simulink model "test_TFOIDFF"  (R2024a)
settings: Solver=VariableStepAuto  StartTime=0.0  StopTime=0.5  RelTol=1e-3
values from neighbouring files (symbols this model uses):
  loadedData = struct()    [colectare_TFOIDFF_simulink.m]
undefined symbols (not defined in the file or in its folder): control_a, control_p, force_a, force_p, minreal, oustapp, rpm_a, rpm_p
libraries: fod x146, slpidlib x15, cstblocks x9
(part 3 of 3)

== system test_TFOIDFF/TFOIDFFID/sensibility/Ord 9 H2 ==
  ref : Inport
  Fractional operator1 : fod/Fractional operator  Tag=Fractional operator  K=96.5  gam=0.99503  ww=[0.001, 1000]  n=7
      settings: SourceProductName=FOMCON Toolbox
  Fractional operator2 : fod/Fractional operator  Tag=Fractional operator  K=-59.619  gam=0.68457  ww=[0.001, 1000]  n=7
      settings: SourceProductName=FOMCON Toolbox
  Fractional operator3 : fod/Fractional operator  Tag=Fractional operator  K=1.4943  gam=0.49298  ww=[0.001, 1000]  n=7
      settings: SourceProductName=FOMCON Toolbox
  Fractional operator4 : fod/Fractional operator  Tag=Fractional operator  K=33.301  gam=0.42823  ww=[0.001, 1000]  n=7
      settings: SourceProductName=FOMCON Toolbox
  Fractional operator5 : fod/Fractional operator  Tag=Fractional operator  K=-67.092  gam=0.40076  ww=[0.001, 1000]  n=7
      settings: SourceProductName=FOMCON Toolbox
  Fractional operator6 : fod/Fractional operator  Tag=Fractional operator  K=55.242  gam=0.29512  ww=[0.001, 1000]  n=7
      settings: SourceProductName=FOMCON Toolbox
  Fractional operator7 : fod/Fractional operator  Tag=Fractional operator  K=53.481  gam=0.25349  ww=[0.001, 1000]  n=7
      settings: SourceProductName=FOMCON Toolbox
  Fractional operator8 : fod/Fractional operator  Tag=Fractional operator  K=42.107  gam=0.15698  ww=[0.001, 1000]  n=7
      settings: SourceProductName=FOMCON Toolbox
  Fractional operator9 : fod/Fractional operator  Tag=Fractional operator  K=-36.49  gam=0.039094  ww=[0.001, 1000]  n=7
      settings: SourceProductName=FOMCON Toolbox
  Sum : Sum  Inputs=|++++++
  Sum1 : Sum  Inputs=|+++
  Sum2 : Sum  Inputs=|++
  comanda : Outport
  wires:
  Sum/1 -> Sum2/1
  ref/1 -> Fractional operator1/1, Fractional operator2/1, Fractional operator9/1, Fractional operator8/1, Fractional operator7/1, Fractional operator6/1, Fractional operator5/1, Fractional operator4/1, Fractional operator3/1
  Fractional operator1/1 -> Sum/1
  Fractional operator2/1 -> Sum/2
  Fractional operator3/1 -> Sum/3
  Fractional operator4/1 -> Sum/4
  Fractional operator5/1 -> Sum/5
  Fractional operator6/1 -> Sum/6
  Fractional operator7/1 -> Sum1/1
  Fractional operator8/1 -> Sum1/2
  Fractional operator9/1 -> Sum1/3
  Sum1/1 -> Sum2/2
  Sum2/1 -> comanda/1

== system test_TFOIDFF/TFOIDFFID/sensibility/Regulator H22 ISE1 ==
  ref : Inport
  Ord 3 : Subsystem
  comanda : Outport
  wires:
  ref/1 -> Ord 3/1(ref)

== system test_TFOIDFF/TFOIDFFID/sensibility/Subsystem ==
  Reg_pitch : Inport
  In2 : Inport  Port=2
  Reg_azimuth : Inport  Port=3
  Azimuth H22 : Gain
  Comanda : Scope  NumInputPorts=3
  Comanda Iesire regulator : Scope  NumInputPorts=2
  D12 : TransferFcn  Numerator=[0.0019343*1 0.0019343*1.287]  Denominator=[1 1.322]
  D21 : TransferFcn  Numerator="[0.0014712*1    0.0014712*3.527]"  Denominator=[1 5.675]
  Pitch H11 : Gain
  Saturation5 : Saturate  UpperLimit=1  LowerLimit=-1  RndMeth=Ceiling
  Saturation6 : Saturate  UpperLimit=1  LowerLimit=-1  RndMeth=Ceiling
  Sum14 : Sum  Inputs=|++
  Sum16 : Sum  Inputs=|++
  TRAS 2_dof model 3 : Subsystem
  azimuth rpm : Outport
  azimuth pos : Outport  Port=2
  pitch rpm : Outport  Port=3
  Comanda1 : Outport  Port=4
  pitch pos : Outport  Port=5
  Comanda2 : Outport  Port=6
  wires:
  TRAS 2_dof model 3/3(rpm_p) -> pitch rpm/1  "pitch rpm"
  Saturation5/1 -> Pitch H11/1  "U_reg_Pitch"
  Azimuth H22/1 -> TRAS 2_dof model 3/1(ctr_a), Comanda1/1  "Comanda"
  TRAS 2_dof model 3/4(pos_p) -> pitch pos/1  "pitch pos"
  Sum14/1 -> Saturation5/1, Comanda Iesire regulator/1  "Pitch"
  Reg_azimuth/1 -> D12/1, Comanda/2, Sum16/2
  Saturation6/1 -> Azimuth H22/1  "U_reg_azimuth"
  TRAS 2_dof model 3/2(pos_a) -> azimuth pos/1  "azimuth pos"
  Pitch H11/1 -> TRAS 2_dof model 3/2(ctr_p), Comanda2/1  "Comanda"
  D12/1 -> Sum14/2
  In2/1 -> Comanda/3
  Sum16/1 -> Saturation6/1, Comanda Iesire regulator/2  "Azimuth"
  Reg_pitch/1 -> D21/1, Sum14/1, Comanda/1
  D21/1 -> Sum16/1
  TRAS 2_dof model 3/1(rpm_a) -> azimuth rpm/1  "azimuth rpm"

== system test_TFOIDFF/TFOIDFFID/IAE/Regulator H22 ISE1/Ord 3 ==
  ref : Inport
  Fractional operator1 : fod/Fractional operator  Tag=Fractional operator  K=97.313  gam=0.98233  ww=[0.001, 1000]  n=7
      settings: SourceProductName=FOMCON Toolbox
  Fractional operator2 : fod/Fractional operator  Tag=Fractional operator  K=44.439  gam=0.76232  ww=[0.001, 1000]  n=7
      settings: SourceProductName=FOMCON Toolbox
  Fractional operator3 : fod/Fractional operator  Tag=Fractional operator  K=-23.784  gam=0.61516  ww=[0.001, 1000]  n=7
      settings: SourceProductName=FOMCON Toolbox
  Sum : Sum  Inputs=+|++
  comanda : Outport
  wires:
  Sum/1 -> comanda/1
  ref/1 -> Fractional operator1/1, Fractional operator2/1, Fractional operator3/1
  Fractional operator1/1 -> Sum/1
  Fractional operator2/1 -> Sum/2
  Fractional operator3/1 -> Sum/3

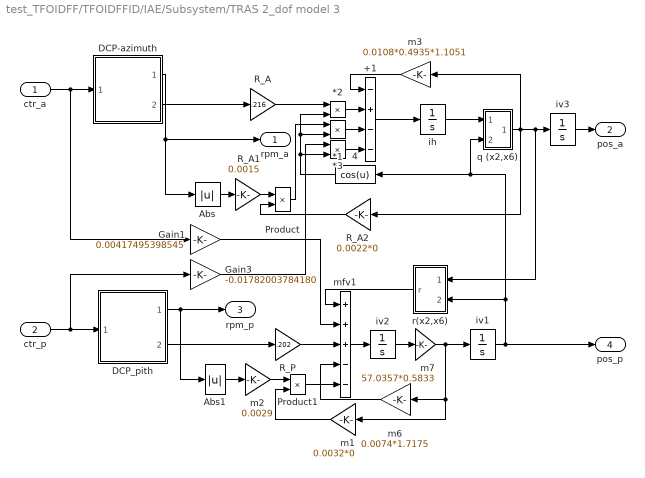
== system test_TFOIDFF/TFOIDFFID/IAE/Subsystem/TRAS 2_dof model 3 ==
  ctr_a : Inport
  ctr_p : Inport  Port=2
  *1 : Product  InputSameDT=on  SaturateOnIntegerOverflow=on  OutDataTypeStr=Inherit: Same as first input
  *2 : Product  InputSameDT=on  SaturateOnIntegerOverflow=on  OutDataTypeStr=Inherit: Same as first input
  *3 : Product  InputSameDT=on  SaturateOnIntegerOverflow=on  OutDataTypeStr=Inherit: Same as first input
  +1 : Sum  Inputs=-+--  InputSameDT=on  SaturateOnIntegerOverflow=on  OutDataTypeStr=Inherit: Same as first input
  4 : Fcn  Expr=cos(u)
  Abs : Abs
  Abs1 : Abs
  DCP-azimuth : Subsystem
  DCP_pith : Subsystem
  Gain1 : Gain  Gain=0.00417495398545  SaturateOnIntegerOverflow=on  OutDataTypeStr=Inherit: Same as input  ParamDataTypeStr=Inherit: Same as input
  Gain3 : Gain  Gain=-0.01782003784180  SaturateOnIntegerOverflow=on  OutDataTypeStr=Inherit: Same as input  ParamDataTypeStr=Inherit: Same as input
  Product : Product  InputSameDT=on  SaturateOnIntegerOverflow=on  OutDataTypeStr=Inherit: Same as first input
  Product1 : Product  SaturateOnIntegerOverflow=on  OutDataTypeStr=Inherit: Same as first input
  R_A : Gain  Gain=.216  OutDataTypeStr=Inherit: Same as input  ParamDataTypeStr=Inherit: Same as input
  R_A1 : Gain  Gain=0.0015  OutDataTypeStr=Inherit: Same as input  ParamDataTypeStr=Inherit: Same as input
  R_A2 : Gain  Gain=0.0022*0  OutDataTypeStr=Inherit: Same as input  ParamDataTypeStr=Inherit: Same as input
  R_P : Gain  Gain=.202  OutDataTypeStr=Inherit: Same as input  ParamDataTypeStr=Inherit: Same as input
  ih : Integrator  UpperSaturationLimit=10  LowerSaturationLimit=-10
  iv1 : Integrator  LimitOutput=on  UpperSaturationLimit=pi/2  LowerSaturationLimit=-pi/2
  iv2 : Integrator  UpperSaturationLimit=pi  LowerSaturationLimit=-pi
  iv3 : Integrator  LimitOutput=on  UpperSaturationLimit=6  LowerSaturationLimit=-6
  m1 : Gain  Gain=0.0032*0  SaturateOnIntegerOverflow=on  OutDataTypeStr=Inherit: Same as input  ParamDataTypeStr=Inherit: Same as input
  m2 : Gain  Gain=0.0029  SaturateOnIntegerOverflow=on  OutDataTypeStr=Inherit: Same as input  ParamDataTypeStr=Inherit: Same as input
  m3 : Gain  Gain=0.0108*0.4935*1.1051  OutDataTypeStr=Inherit: Same as input  ParamDataTypeStr=Inherit: Same as input
  m6 : Gain  Gain=0.0074*1.7175  OutDataTypeStr=Inherit: Same as input  ParamDataTypeStr=Inherit: Same as input
  m7 : Gain  Gain=57.0357*0.5833  SaturateOnIntegerOverflow=on  OutDataTypeStr=Inherit: Same as input  ParamDataTypeStr=Inherit: Same as input
  mfv1 : Sum  Inputs=+++--  InputSameDT=on  SaturateOnIntegerOverflow=on  OutDataTypeStr=Inherit: Same as first input
  q (x2,x6) : Subsystem
  r(x2,x6) : Subsystem
  rpm_a : Outport
  pos_a : Outport  Port=2
  rpm_p : Outport  Port=3
  pos_p : Outport  Port=4
  wires:
  DCP-azimuth/1(RPM_A) -> Abs/1, rpm_a/1
  +1/1 -> ih/1
  iv3/1 -> pos_a/1
  ctr_p/1 -> Gain3/1, DCP_pith/1(CTR_P)
  ctr_a/1 -> Gain1/1, DCP-azimuth/1(CTR_A)
  Gain3/1 -> *3/1
  Gain1/1 -> mfv1/2
  4/1 -> *3/2, *1/2, *2/2
  Product/1 -> *1/1
  *3/1 -> +1/4
  m2/1 -> Product1/1
  m1/1 -> Product1/2
  iv1/1 -> q (x2,x6)/2(x6), 4/1, r(x2,x6)/2(x6), pos_p/1
  R_P/1 -> mfv1/3
  r(x2,x6)/1(r) -> mfv1/1
  Product1/1 -> mfv1/5
  Abs1/1 -> m2/1
  DCP_pith/1(RPM_P) -> rpm_p/1, Abs1/1
  m7/1 -> m6/1, m1/1, iv1/1
  mfv1/1 -> iv2/1
  iv2/1 -> m7/1
  m6/1 -> mfv1/4
  DCP_pith/2(FORCE_P) -> R_P/1
  R_A2/1 -> Product/2
  R_A1/1 -> Product/1
  Abs/1 -> R_A1/1
  R_A/1 -> *2/1
  q (x2,x6)/1(q) -> R_A2/1, m3/1, r(x2,x6)/1(y2), iv3/1
  ih/1 -> q (x2,x6)/1(x2)
  *2/1 -> +1/2
  m3/1 -> +1/1
  *1/1 -> +1/3
  DCP-azimuth/2(FORCE_A) -> R_A/1

== system test_TFOIDFF/TFOIDFFID/ISE/Regulator H22 ISE1/Ord 3 ==
  ref : Inport
  Fractional operator1 : fod/Fractional operator  Tag=Fractional operator  K=97.313  gam=0.98233  ww=[0.001, 1000]  n=7
      settings: SourceProductName=FOMCON Toolbox
  Fractional operator2 : fod/Fractional operator  Tag=Fractional operator  K=44.439  gam=0.76232  ww=[0.001, 1000]  n=7
      settings: SourceProductName=FOMCON Toolbox
  Fractional operator3 : fod/Fractional operator  Tag=Fractional operator  K=-23.784  gam=0.61516  ww=[0.001, 1000]  n=7
      settings: SourceProductName=FOMCON Toolbox
  Sum : Sum  Inputs=+|++
  comanda : Outport
  wires:
  Sum/1 -> comanda/1
  ref/1 -> Fractional operator1/1, Fractional operator2/1, Fractional operator3/1
  Fractional operator1/1 -> Sum/1
  Fractional operator2/1 -> Sum/2
  Fractional operator3/1 -> Sum/3

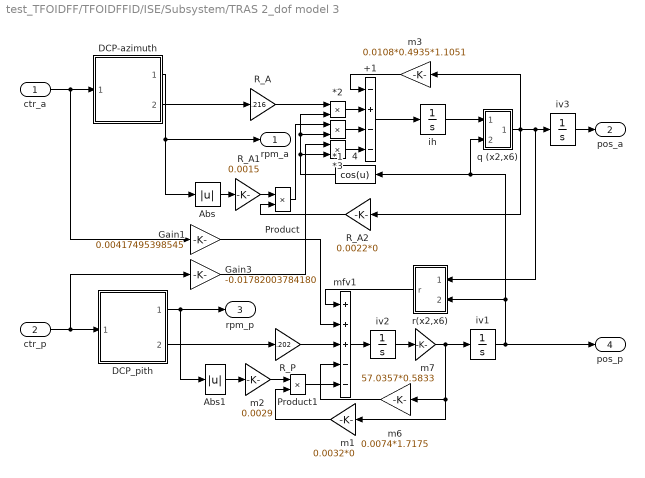
== system test_TFOIDFF/TFOIDFFID/ISE/Subsystem/TRAS 2_dof model 3 ==
  ctr_a : Inport
  ctr_p : Inport  Port=2
  *1 : Product  InputSameDT=on  SaturateOnIntegerOverflow=on  OutDataTypeStr=Inherit: Same as first input
  *2 : Product  InputSameDT=on  SaturateOnIntegerOverflow=on  OutDataTypeStr=Inherit: Same as first input
  *3 : Product  InputSameDT=on  SaturateOnIntegerOverflow=on  OutDataTypeStr=Inherit: Same as first input
  +1 : Sum  Inputs=-+--  InputSameDT=on  SaturateOnIntegerOverflow=on  OutDataTypeStr=Inherit: Same as first input
  4 : Fcn  Expr=cos(u)
  Abs : Abs
  Abs1 : Abs
  DCP-azimuth : Subsystem
  DCP_pith : Subsystem
  Gain1 : Gain  Gain=0.00417495398545  SaturateOnIntegerOverflow=on  OutDataTypeStr=Inherit: Same as input  ParamDataTypeStr=Inherit: Same as input
  Gain3 : Gain  Gain=-0.01782003784180  SaturateOnIntegerOverflow=on  OutDataTypeStr=Inherit: Same as input  ParamDataTypeStr=Inherit: Same as input
  Product : Product  InputSameDT=on  SaturateOnIntegerOverflow=on  OutDataTypeStr=Inherit: Same as first input
  Product1 : Product  SaturateOnIntegerOverflow=on  OutDataTypeStr=Inherit: Same as first input
  R_A : Gain  Gain=.216  OutDataTypeStr=Inherit: Same as input  ParamDataTypeStr=Inherit: Same as input
  R_A1 : Gain  Gain=0.0015  OutDataTypeStr=Inherit: Same as input  ParamDataTypeStr=Inherit: Same as input
  R_A2 : Gain  Gain=0.0022*0  OutDataTypeStr=Inherit: Same as input  ParamDataTypeStr=Inherit: Same as input
  R_P : Gain  Gain=.202  OutDataTypeStr=Inherit: Same as input  ParamDataTypeStr=Inherit: Same as input
  ih : Integrator  UpperSaturationLimit=10  LowerSaturationLimit=-10
  iv1 : Integrator  LimitOutput=on  UpperSaturationLimit=pi/2  LowerSaturationLimit=-pi/2
  iv2 : Integrator  UpperSaturationLimit=pi  LowerSaturationLimit=-pi
  iv3 : Integrator  LimitOutput=on  UpperSaturationLimit=6  LowerSaturationLimit=-6
  m1 : Gain  Gain=0.0032*0  SaturateOnIntegerOverflow=on  OutDataTypeStr=Inherit: Same as input  ParamDataTypeStr=Inherit: Same as input
  m2 : Gain  Gain=0.0029  SaturateOnIntegerOverflow=on  OutDataTypeStr=Inherit: Same as input  ParamDataTypeStr=Inherit: Same as input
  m3 : Gain  Gain=0.0108*0.4935*1.1051  OutDataTypeStr=Inherit: Same as input  ParamDataTypeStr=Inherit: Same as input
  m6 : Gain  Gain=0.0074*1.7175  OutDataTypeStr=Inherit: Same as input  ParamDataTypeStr=Inherit: Same as input
  m7 : Gain  Gain=57.0357*0.5833  SaturateOnIntegerOverflow=on  OutDataTypeStr=Inherit: Same as input  ParamDataTypeStr=Inherit: Same as input
  mfv1 : Sum  Inputs=+++--  InputSameDT=on  SaturateOnIntegerOverflow=on  OutDataTypeStr=Inherit: Same as first input
  q (x2,x6) : Subsystem
  r(x2,x6) : Subsystem
  rpm_a : Outport
  pos_a : Outport  Port=2
  rpm_p : Outport  Port=3
  pos_p : Outport  Port=4
  wires:
  DCP-azimuth/1(RPM_A) -> Abs/1, rpm_a/1
  +1/1 -> ih/1
  iv3/1 -> pos_a/1
  ctr_p/1 -> Gain3/1, DCP_pith/1(CTR_P)
  ctr_a/1 -> Gain1/1, DCP-azimuth/1(CTR_A)
  Gain3/1 -> *3/1
  Gain1/1 -> mfv1/2
  4/1 -> *3/2, *1/2, *2/2
  Product/1 -> *1/1
  *3/1 -> +1/4
  m2/1 -> Product1/1
  m1/1 -> Product1/2
  iv1/1 -> q (x2,x6)/2(x6), 4/1, r(x2,x6)/2(x6), pos_p/1
  R_P/1 -> mfv1/3
  r(x2,x6)/1(r) -> mfv1/1
  Product1/1 -> mfv1/5
  Abs1/1 -> m2/1
  DCP_pith/1(RPM_P) -> rpm_p/1, Abs1/1
  m7/1 -> m6/1, m1/1, iv1/1
  mfv1/1 -> iv2/1
  iv2/1 -> m7/1
  m6/1 -> mfv1/4
  DCP_pith/2(FORCE_P) -> R_P/1
  R_A2/1 -> Product/2
  R_A1/1 -> Product/1
  Abs/1 -> R_A1/1
  R_A/1 -> *2/1
  q (x2,x6)/1(q) -> R_A2/1, m3/1, r(x2,x6)/1(y2), iv3/1
  ih/1 -> q (x2,x6)/1(x2)
  *2/1 -> +1/2
  m3/1 -> +1/1
  *1/1 -> +1/3
  DCP-azimuth/2(FORCE_A) -> R_A/1

== system test_TFOIDFF/TFOIDFFID/ITAE/Regulator H22 ISE1/Ord 3 ==
  ref : Inport
  Fractional operator1 : fod/Fractional operator  Tag=Fractional operator  K=97.313  gam=0.98233  ww=[0.001, 1000]  n=7
      settings: SourceProductName=FOMCON Toolbox
  Fractional operator2 : fod/Fractional operator  Tag=Fractional operator  K=44.439  gam=0.76232  ww=[0.001, 1000]  n=7
      settings: SourceProductName=FOMCON Toolbox
  Fractional operator3 : fod/Fractional operator  Tag=Fractional operator  K=-23.784  gam=0.61516  ww=[0.001, 1000]  n=7
      settings: SourceProductName=FOMCON Toolbox
  Sum : Sum  Inputs=+|++
  comanda : Outport
  wires:
  Fractional operator3/1 -> Sum/3
  Fractional operator2/1 -> Sum/2
  Fractional operator1/1 -> Sum/1
  ref/1 -> Fractional operator3/1, Fractional operator2/1, Fractional operator1/1
  Sum/1 -> comanda/1

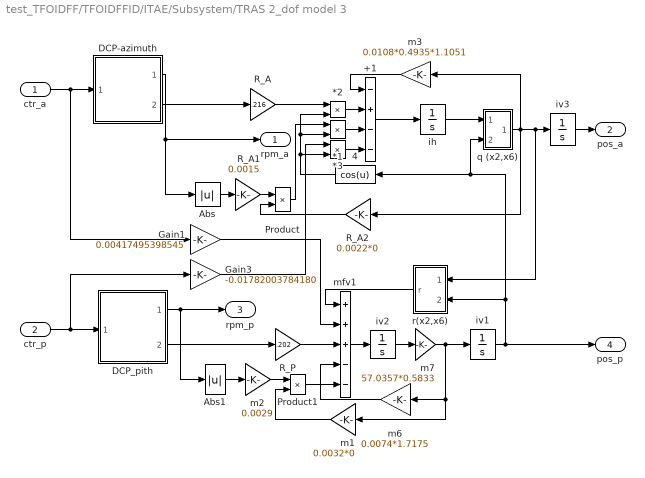
== system test_TFOIDFF/TFOIDFFID/ITAE/Subsystem/TRAS 2_dof model 3 ==
  ctr_a : Inport
  ctr_p : Inport  Port=2
  *1 : Product  InputSameDT=on  SaturateOnIntegerOverflow=on  OutDataTypeStr=Inherit: Same as first input
  *2 : Product  InputSameDT=on  SaturateOnIntegerOverflow=on  OutDataTypeStr=Inherit: Same as first input
  *3 : Product  InputSameDT=on  SaturateOnIntegerOverflow=on  OutDataTypeStr=Inherit: Same as first input
  +1 : Sum  Inputs=-+--  InputSameDT=on  SaturateOnIntegerOverflow=on  OutDataTypeStr=Inherit: Same as first input
  4 : Fcn  Expr=cos(u)
  Abs : Abs
  Abs1 : Abs
  DCP-azimuth : Subsystem
  DCP_pith : Subsystem
  Gain1 : Gain  Gain=0.00417495398545  SaturateOnIntegerOverflow=on  OutDataTypeStr=Inherit: Same as input  ParamDataTypeStr=Inherit: Same as input
  Gain3 : Gain  Gain=-0.01782003784180  SaturateOnIntegerOverflow=on  OutDataTypeStr=Inherit: Same as input  ParamDataTypeStr=Inherit: Same as input
  Product : Product  InputSameDT=on  SaturateOnIntegerOverflow=on  OutDataTypeStr=Inherit: Same as first input
  Product1 : Product  SaturateOnIntegerOverflow=on  OutDataTypeStr=Inherit: Same as first input
  R_A : Gain  Gain=.216  OutDataTypeStr=Inherit: Same as input  ParamDataTypeStr=Inherit: Same as input
  R_A1 : Gain  Gain=0.0015  OutDataTypeStr=Inherit: Same as input  ParamDataTypeStr=Inherit: Same as input
  R_A2 : Gain  Gain=0.0022*0  OutDataTypeStr=Inherit: Same as input  ParamDataTypeStr=Inherit: Same as input
  R_P : Gain  Gain=.202  OutDataTypeStr=Inherit: Same as input  ParamDataTypeStr=Inherit: Same as input
  ih : Integrator  UpperSaturationLimit=10  LowerSaturationLimit=-10
  iv1 : Integrator  LimitOutput=on  UpperSaturationLimit=pi/2  LowerSaturationLimit=-pi/2
  iv2 : Integrator  UpperSaturationLimit=pi  LowerSaturationLimit=-pi
  iv3 : Integrator  LimitOutput=on  UpperSaturationLimit=6  LowerSaturationLimit=-6
  m1 : Gain  Gain=0.0032*0  SaturateOnIntegerOverflow=on  OutDataTypeStr=Inherit: Same as input  ParamDataTypeStr=Inherit: Same as input
  m2 : Gain  Gain=0.0029  SaturateOnIntegerOverflow=on  OutDataTypeStr=Inherit: Same as input  ParamDataTypeStr=Inherit: Same as input
  m3 : Gain  Gain=0.0108*0.4935*1.1051  OutDataTypeStr=Inherit: Same as input  ParamDataTypeStr=Inherit: Same as input
  m6 : Gain  Gain=0.0074*1.7175  OutDataTypeStr=Inherit: Same as input  ParamDataTypeStr=Inherit: Same as input
  m7 : Gain  Gain=57.0357*0.5833  SaturateOnIntegerOverflow=on  OutDataTypeStr=Inherit: Same as input  ParamDataTypeStr=Inherit: Same as input
  mfv1 : Sum  Inputs=+++--  InputSameDT=on  SaturateOnIntegerOverflow=on  OutDataTypeStr=Inherit: Same as first input
  q (x2,x6) : Subsystem
  r(x2,x6) : Subsystem
  rpm_a : Outport
  pos_a : Outport  Port=2
  rpm_p : Outport  Port=3
  pos_p : Outport  Port=4
  wires:
  DCP-azimuth/2(FORCE_A) -> R_A/1
  *1/1 -> +1/3
  m3/1 -> +1/1
  *2/1 -> +1/2
  ih/1 -> q (x2,x6)/1(x2)
  q (x2,x6)/1(q) -> iv3/1, r(x2,x6)/1(y2), m3/1, R_A2/1
  R_A/1 -> *2/1
  Abs/1 -> R_A1/1
  R_A1/1 -> Product/1
  R_A2/1 -> Product/2
  DCP_pith/2(FORCE_P) -> R_P/1
  m6/1 -> mfv1/4
  iv2/1 -> m7/1
  mfv1/1 -> iv2/1
  m7/1 -> iv1/1, m1/1, m6/1
  DCP_pith/1(RPM_P) -> Abs1/1, rpm_p/1
  Abs1/1 -> m2/1
  Product1/1 -> mfv1/5
  r(x2,x6)/1(r) -> mfv1/1
  R_P/1 -> mfv1/3
  iv1/1 -> pos_p/1, r(x2,x6)/2(x6), 4/1, q (x2,x6)/2(x6)
  m1/1 -> Product1/2
  m2/1 -> Product1/1
  *3/1 -> +1/4
  Product/1 -> *1/1
  4/1 -> *2/2, *1/2, *3/2
  Gain1/1 -> mfv1/2
  Gain3/1 -> *3/1
  ctr_a/1 -> DCP-azimuth/1(CTR_A), Gain1/1
  ctr_p/1 -> DCP_pith/1(CTR_P), Gain3/1
  iv3/1 -> pos_a/1
  +1/1 -> ih/1
  DCP-azimuth/1(RPM_A) -> rpm_a/1, Abs/1

== system test_TFOIDFF/TFOIDFFID/ITSE/Regulator H22 ISE1/Ord 3 ==
  ref : Inport
  Fractional operator1 : fod/Fractional operator  Tag=Fractional operator  K=97.313  gam=0.98233  ww=[0.001, 1000]  n=7
      settings: SourceProductName=FOMCON Toolbox
  Fractional operator2 : fod/Fractional operator  Tag=Fractional operator  K=44.439  gam=0.76232  ww=[0.001, 1000]  n=7
      settings: SourceProductName=FOMCON Toolbox
  Fractional operator3 : fod/Fractional operator  Tag=Fractional operator  K=-23.784  gam=0.61516  ww=[0.001, 1000]  n=7
      settings: SourceProductName=FOMCON Toolbox
  Sum : Sum  Inputs=+|++
  comanda : Outport
  wires:
  Fractional operator3/1 -> Sum/3
  Fractional operator2/1 -> Sum/2
  Fractional operator1/1 -> Sum/1
  ref/1 -> Fractional operator3/1, Fractional operator2/1, Fractional operator1/1
  Sum/1 -> comanda/1

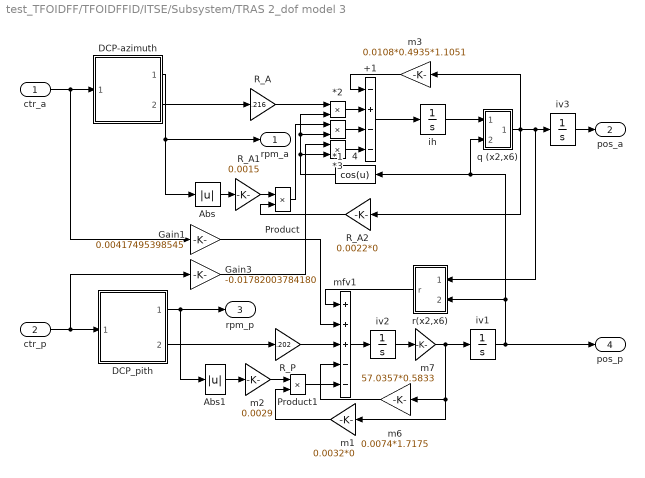
== system test_TFOIDFF/TFOIDFFID/ITSE/Subsystem/TRAS 2_dof model 3 ==
  ctr_a : Inport
  ctr_p : Inport  Port=2
  *1 : Product  InputSameDT=on  SaturateOnIntegerOverflow=on  OutDataTypeStr=Inherit: Same as first input
  *2 : Product  InputSameDT=on  SaturateOnIntegerOverflow=on  OutDataTypeStr=Inherit: Same as first input
  *3 : Product  InputSameDT=on  SaturateOnIntegerOverflow=on  OutDataTypeStr=Inherit: Same as first input
  +1 : Sum  Inputs=-+--  InputSameDT=on  SaturateOnIntegerOverflow=on  OutDataTypeStr=Inherit: Same as first input
  4 : Fcn  Expr=cos(u)
  Abs : Abs
  Abs1 : Abs
  DCP-azimuth : Subsystem
  DCP_pith : Subsystem
  Gain1 : Gain  Gain=0.00417495398545  SaturateOnIntegerOverflow=on  OutDataTypeStr=Inherit: Same as input  ParamDataTypeStr=Inherit: Same as input
  Gain3 : Gain  Gain=-0.01782003784180  SaturateOnIntegerOverflow=on  OutDataTypeStr=Inherit: Same as input  ParamDataTypeStr=Inherit: Same as input
  Product : Product  InputSameDT=on  SaturateOnIntegerOverflow=on  OutDataTypeStr=Inherit: Same as first input
  Product1 : Product  SaturateOnIntegerOverflow=on  OutDataTypeStr=Inherit: Same as first input
  R_A : Gain  Gain=.216  OutDataTypeStr=Inherit: Same as input  ParamDataTypeStr=Inherit: Same as input
  R_A1 : Gain  Gain=0.0015  OutDataTypeStr=Inherit: Same as input  ParamDataTypeStr=Inherit: Same as input
  R_A2 : Gain  Gain=0.0022*0  OutDataTypeStr=Inherit: Same as input  ParamDataTypeStr=Inherit: Same as input
  R_P : Gain  Gain=.202  OutDataTypeStr=Inherit: Same as input  ParamDataTypeStr=Inherit: Same as input
  ih : Integrator  UpperSaturationLimit=10  LowerSaturationLimit=-10
  iv1 : Integrator  LimitOutput=on  UpperSaturationLimit=pi/2  LowerSaturationLimit=-pi/2
  iv2 : Integrator  UpperSaturationLimit=pi  LowerSaturationLimit=-pi
  iv3 : Integrator  LimitOutput=on  UpperSaturationLimit=6  LowerSaturationLimit=-6
  m1 : Gain  Gain=0.0032*0  SaturateOnIntegerOverflow=on  OutDataTypeStr=Inherit: Same as input  ParamDataTypeStr=Inherit: Same as input
  m2 : Gain  Gain=0.0029  SaturateOnIntegerOverflow=on  OutDataTypeStr=Inherit: Same as input  ParamDataTypeStr=Inherit: Same as input
  m3 : Gain  Gain=0.0108*0.4935*1.1051  OutDataTypeStr=Inherit: Same as input  ParamDataTypeStr=Inherit: Same as input
  m6 : Gain  Gain=0.0074*1.7175  OutDataTypeStr=Inherit: Same as input  ParamDataTypeStr=Inherit: Same as input
  m7 : Gain  Gain=57.0357*0.5833  SaturateOnIntegerOverflow=on  OutDataTypeStr=Inherit: Same as input  ParamDataTypeStr=Inherit: Same as input
  mfv1 : Sum  Inputs=+++--  InputSameDT=on  SaturateOnIntegerOverflow=on  OutDataTypeStr=Inherit: Same as first input
  q (x2,x6) : Subsystem
  r(x2,x6) : Subsystem
  rpm_a : Outport
  pos_a : Outport  Port=2
  rpm_p : Outport  Port=3
  pos_p : Outport  Port=4
  wires:
  DCP-azimuth/2(FORCE_A) -> R_A/1
  *1/1 -> +1/3
  m3/1 -> +1/1
  *2/1 -> +1/2
  ih/1 -> q (x2,x6)/1(x2)
  q (x2,x6)/1(q) -> iv3/1, r(x2,x6)/1(y2), m3/1, R_A2/1
  R_A/1 -> *2/1
  Abs/1 -> R_A1/1
  R_A1/1 -> Product/1
  R_A2/1 -> Product/2
  DCP_pith/2(FORCE_P) -> R_P/1
  m6/1 -> mfv1/4
  iv2/1 -> m7/1
  mfv1/1 -> iv2/1
  m7/1 -> iv1/1, m1/1, m6/1
  DCP_pith/1(RPM_P) -> Abs1/1, rpm_p/1
  Abs1/1 -> m2/1
  Product1/1 -> mfv1/5
  r(x2,x6)/1(r) -> mfv1/1
  R_P/1 -> mfv1/3
  iv1/1 -> pos_p/1, r(x2,x6)/2(x6), 4/1, q (x2,x6)/2(x6)
  m1/1 -> Product1/2
  m2/1 -> Product1/1
  *3/1 -> +1/4
  Product/1 -> *1/1
  4/1 -> *2/2, *1/2, *3/2
  Gain1/1 -> mfv1/2
  Gain3/1 -> *3/1
  ctr_a/1 -> DCP-azimuth/1(CTR_A), Gain1/1
  ctr_p/1 -> DCP_pith/1(CTR_P), Gain3/1
  iv3/1 -> pos_a/1
  +1/1 -> ih/1
  DCP-azimuth/1(RPM_A) -> rpm_a/1, Abs/1

== system test_TFOIDFF/TFOIDFFID/sensibility/Regulator H22 ISE1/Ord 3 ==
  ref : Inport
  Fractional operator1 : fod/Fractional operator  Tag=Fractional operator  K=97.313  gam=0.98233  ww=[0.001, 1000]  n=7
      settings: SourceProductName=FOMCON Toolbox
  Fractional operator2 : fod/Fractional operator  Tag=Fractional operator  K=44.439  gam=0.76232  ww=[0.001, 1000]  n=7
      settings: SourceProductName=FOMCON Toolbox
  Fractional operator3 : fod/Fractional operator  Tag=Fractional operator  K=-23.784  gam=0.61516  ww=[0.001, 1000]  n=7
      settings: SourceProductName=FOMCON Toolbox
  Sum : Sum  Inputs=+|++
  comanda : Outport
  wires:
  Sum/1 -> comanda/1
  ref/1 -> Fractional operator1/1, Fractional operator2/1, Fractional operator3/1
  Fractional operator1/1 -> Sum/1
  Fractional operator2/1 -> Sum/2
  Fractional operator3/1 -> Sum/3

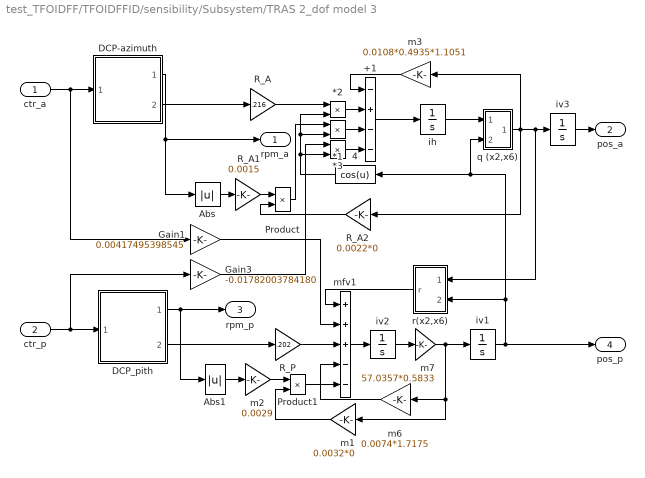
== system test_TFOIDFF/TFOIDFFID/sensibility/Subsystem/TRAS 2_dof model 3 ==
  ctr_a : Inport
  ctr_p : Inport  Port=2
  *1 : Product  InputSameDT=on  SaturateOnIntegerOverflow=on  OutDataTypeStr=Inherit: Same as first input
  *2 : Product  InputSameDT=on  SaturateOnIntegerOverflow=on  OutDataTypeStr=Inherit: Same as first input
  *3 : Product  InputSameDT=on  SaturateOnIntegerOverflow=on  OutDataTypeStr=Inherit: Same as first input
  +1 : Sum  Inputs=-+--  InputSameDT=on  SaturateOnIntegerOverflow=on  OutDataTypeStr=Inherit: Same as first input
  4 : Fcn  Expr=cos(u)
  Abs : Abs
  Abs1 : Abs
  DCP-azimuth : Subsystem
  DCP_pith : Subsystem
  Gain1 : Gain  Gain=0.00417495398545  SaturateOnIntegerOverflow=on  OutDataTypeStr=Inherit: Same as input  ParamDataTypeStr=Inherit: Same as input
  Gain3 : Gain  Gain=-0.01782003784180  SaturateOnIntegerOverflow=on  OutDataTypeStr=Inherit: Same as input  ParamDataTypeStr=Inherit: Same as input
  Product : Product  InputSameDT=on  SaturateOnIntegerOverflow=on  OutDataTypeStr=Inherit: Same as first input
  Product1 : Product  SaturateOnIntegerOverflow=on  OutDataTypeStr=Inherit: Same as first input
  R_A : Gain  Gain=.216  OutDataTypeStr=Inherit: Same as input  ParamDataTypeStr=Inherit: Same as input
  R_A1 : Gain  Gain=0.0015  OutDataTypeStr=Inherit: Same as input  ParamDataTypeStr=Inherit: Same as input
  R_A2 : Gain  Gain=0.0022*0  OutDataTypeStr=Inherit: Same as input  ParamDataTypeStr=Inherit: Same as input
  R_P : Gain  Gain=.202  OutDataTypeStr=Inherit: Same as input  ParamDataTypeStr=Inherit: Same as input
  ih : Integrator  UpperSaturationLimit=10  LowerSaturationLimit=-10
  iv1 : Integrator  LimitOutput=on  UpperSaturationLimit=pi/2  LowerSaturationLimit=-pi/2
  iv2 : Integrator  UpperSaturationLimit=pi  LowerSaturationLimit=-pi
  iv3 : Integrator  LimitOutput=on  UpperSaturationLimit=6  LowerSaturationLimit=-6
  m1 : Gain  Gain=0.0032*0  SaturateOnIntegerOverflow=on  OutDataTypeStr=Inherit: Same as input  ParamDataTypeStr=Inherit: Same as input
  m2 : Gain  Gain=0.0029  SaturateOnIntegerOverflow=on  OutDataTypeStr=Inherit: Same as input  ParamDataTypeStr=Inherit: Same as input
  m3 : Gain  Gain=0.0108*0.4935*1.1051  OutDataTypeStr=Inherit: Same as input  ParamDataTypeStr=Inherit: Same as input
  m6 : Gain  Gain=0.0074*1.7175  OutDataTypeStr=Inherit: Same as input  ParamDataTypeStr=Inherit: Same as input
  m7 : Gain  Gain=57.0357*0.5833  SaturateOnIntegerOverflow=on  OutDataTypeStr=Inherit: Same as input  ParamDataTypeStr=Inherit: Same as input
  mfv1 : Sum  Inputs=+++--  InputSameDT=on  SaturateOnIntegerOverflow=on  OutDataTypeStr=Inherit: Same as first input
  q (x2,x6) : Subsystem
  r(x2,x6) : Subsystem
  rpm_a : Outport
  pos_a : Outport  Port=2
  rpm_p : Outport  Port=3
  pos_p : Outport  Port=4
  wires:
  DCP-azimuth/1(RPM_A) -> Abs/1, rpm_a/1
  +1/1 -> ih/1
  iv3/1 -> pos_a/1
  ctr_p/1 -> Gain3/1, DCP_pith/1(CTR_P)
  ctr_a/1 -> Gain1/1, DCP-azimuth/1(CTR_A)
  Gain3/1 -> *3/1
  Gain1/1 -> mfv1/2
  4/1 -> *3/2, *1/2, *2/2
  Product/1 -> *1/1
  *3/1 -> +1/4
  m2/1 -> Product1/1
  m1/1 -> Product1/2
  iv1/1 -> q (x2,x6)/2(x6), 4/1, r(x2,x6)/2(x6), pos_p/1
  R_P/1 -> mfv1/3
  r(x2,x6)/1(r) -> mfv1/1
  Product1/1 -> mfv1/5
  Abs1/1 -> m2/1
  DCP_pith/1(RPM_P) -> rpm_p/1, Abs1/1
  m7/1 -> m6/1, m1/1, iv1/1
  mfv1/1 -> iv2/1
  iv2/1 -> m7/1
  m6/1 -> mfv1/4
  DCP_pith/2(FORCE_P) -> R_P/1
  R_A2/1 -> Product/2
  R_A1/1 -> Product/1
  Abs/1 -> R_A1/1
  R_A/1 -> *2/1
  q (x2,x6)/1(q) -> R_A2/1, m3/1, r(x2,x6)/1(y2), iv3/1
  ih/1 -> q (x2,x6)/1(x2)
  *2/1 -> +1/2
  m3/1 -> +1/1
  *1/1 -> +1/3
  DCP-azimuth/2(FORCE_A) -> R_A/1

== system test_TFOIDFF/TFOIDFFID/IAE/Subsystem/TRAS 2_dof model 3/DCP-azimuth ==
  CTR_A : Inport
  1/Ja : Gain  Gain=37000  SaturateOnIntegerOverflow=on  OutDataTypeStr=Inherit: Same as input  ParamDataTypeStr=Inherit: Same as input
  CtrlA(rpma) : Lookup  InputValues=rpm_a  Table=control_a
  Integrator1 : Integrator
  Sum1 : Sum  Inputs=|+-  InputSameDT=on  SaturateOnIntegerOverflow=on  OutDataTypeStr=Inherit: Same as first input
  forceA(rpma) : Lookup  InputValues=rpm_a  Table=force_a
  RPM_A : Outport
  FORCE_A : Outport  Port=2
  wires:
  forceA(rpma)/1 -> FORCE_A/1
  CTR_A/1 -> Sum1/1
  1/Ja/1 -> RPM_A/1, forceA(rpma)/1, CtrlA(rpma)/1
  Integrator1/1 -> 1/Ja/1
  CtrlA(rpma)/1 -> Sum1/2
  Sum1/1 -> Integrator1/1

== system test_TFOIDFF/TFOIDFFID/IAE/Subsystem/TRAS 2_dof model 3/DCP_pith ==
  CTR_P : Inport
  1/Jp1 : Gain  Gain=6100  OutDataTypeStr=Inherit: Same as input  ParamDataTypeStr=Inherit: Same as input
  CtrlP(rpmp) : Lookup  InputValues=rpm_p  Table=control_p
  Integrator : Integrator
  Sum : Sum  Inputs=|+-  InputSameDT=on  SaturateOnIntegerOverflow=on  OutDataTypeStr=Inherit: Same as first input
  force(rpmp) : Lookup  InputValues=rpm_p  Table=force_p
  RPM_P : Outport
  FORCE_P : Outport  Port=2
  wires:
  force(rpmp)/1 -> FORCE_P/1
  CTR_P/1 -> Sum/1
  1/Jp1/1 -> force(rpmp)/1, CtrlP(rpmp)/1, RPM_P/1
  CtrlP(rpmp)/1 -> Sum/2
  Integrator/1 -> 1/Jp1/1
  Sum/1 -> Integrator/1

== system test_TFOIDFF/TFOIDFFID/IAE/Subsystem/TRAS 2_dof model 3/q (x2,x6) ==
  x2 : Inport
  x6 : Inport  Port=2
  " q(x6)" : Fcn  Expr=( (0.0268-0.00300962066650)*cos(u)^2) +0.00300962066650
  *1 : Product  Inputs=*/  InputSameDT=on  SaturateOnIntegerOverflow=on  OutDataTypeStr=Inherit: Same as first input
  q : Outport
  wires:
  " q(x6)"/1 -> *1/2
  x6/1 -> " q(x6)"/1
  x2/1 -> *1/1
  *1/1 -> q/1

== system test_TFOIDFF/TFOIDFFID/IAE/Subsystem/TRAS 2_dof model 3/r(x2,x6) ==
  y2 : Inport
  x6 : Inport  Port=2
  +2 : Sum  InputSameDT=on  SaturateOnIntegerOverflow=on  OutDataTypeStr=Inherit: Same as first input
  Mux : Mux  Inputs=2
  r2 : Fcn  Expr=- ( 0.0292*cos(u)+ 0.0546*sin(u))*1.7143
  s : Fcn  Expr="(u(1)^2)*(     -0.07389953104162*  0.28753198180218*sin(u(2))*cos(u(2)))"
  r : Outport
  wires:
  y2/1 -> Mux/1
  +2/1 -> r/1
  x6/1 -> r2/1, Mux/2
  s/1 -> +2/2
  r2/1 -> +2/1
  Mux/1 -> s/1

== system test_TFOIDFF/TFOIDFFID/ISE/Subsystem/TRAS 2_dof model 3/DCP-azimuth ==
  CTR_A : Inport
  1/Ja : Gain  Gain=37000  SaturateOnIntegerOverflow=on  OutDataTypeStr=Inherit: Same as input  ParamDataTypeStr=Inherit: Same as input
  CtrlA(rpma) : Lookup  InputValues=rpm_a  Table=control_a
  Integrator1 : Integrator
  Sum1 : Sum  Inputs=|+-  InputSameDT=on  SaturateOnIntegerOverflow=on  OutDataTypeStr=Inherit: Same as first input
  forceA(rpma) : Lookup  InputValues=rpm_a  Table=force_a
  RPM_A : Outport
  FORCE_A : Outport  Port=2
  wires:
  forceA(rpma)/1 -> FORCE_A/1
  CTR_A/1 -> Sum1/1
  1/Ja/1 -> RPM_A/1, forceA(rpma)/1, CtrlA(rpma)/1
  Integrator1/1 -> 1/Ja/1
  CtrlA(rpma)/1 -> Sum1/2
  Sum1/1 -> Integrator1/1

== system test_TFOIDFF/TFOIDFFID/ISE/Subsystem/TRAS 2_dof model 3/DCP_pith ==
  CTR_P : Inport
  1/Jp1 : Gain  Gain=6100  OutDataTypeStr=Inherit: Same as input  ParamDataTypeStr=Inherit: Same as input
  CtrlP(rpmp) : Lookup  InputValues=rpm_p  Table=control_p
  Integrator : Integrator
  Sum : Sum  Inputs=|+-  InputSameDT=on  SaturateOnIntegerOverflow=on  OutDataTypeStr=Inherit: Same as first input
  force(rpmp) : Lookup  InputValues=rpm_p  Table=force_p
  RPM_P : Outport
  FORCE_P : Outport  Port=2
  wires:
  force(rpmp)/1 -> FORCE_P/1
  CTR_P/1 -> Sum/1
  1/Jp1/1 -> force(rpmp)/1, CtrlP(rpmp)/1, RPM_P/1
  CtrlP(rpmp)/1 -> Sum/2
  Integrator/1 -> 1/Jp1/1
  Sum/1 -> Integrator/1

== system test_TFOIDFF/TFOIDFFID/ISE/Subsystem/TRAS 2_dof model 3/q (x2,x6) ==
  x2 : Inport
  x6 : Inport  Port=2
  " q(x6)" : Fcn  Expr=( (0.0268-0.00300962066650)*cos(u)^2) +0.00300962066650
  *1 : Product  Inputs=*/  InputSameDT=on  SaturateOnIntegerOverflow=on  OutDataTypeStr=Inherit: Same as first input
  q : Outport
  wires:
  " q(x6)"/1 -> *1/2
  x6/1 -> " q(x6)"/1
  x2/1 -> *1/1
  *1/1 -> q/1

== system test_TFOIDFF/TFOIDFFID/ISE/Subsystem/TRAS 2_dof model 3/r(x2,x6) ==
  y2 : Inport
  x6 : Inport  Port=2
  +2 : Sum  InputSameDT=on  SaturateOnIntegerOverflow=on  OutDataTypeStr=Inherit: Same as first input
  Mux : Mux  Inputs=2
  r2 : Fcn  Expr=- ( 0.0292*cos(u)+ 0.0546*sin(u))*1.7143
  s : Fcn  Expr="(u(1)^2)*(     -0.07389953104162*  0.28753198180218*sin(u(2))*cos(u(2)))"
  r : Outport
  wires:
  y2/1 -> Mux/1
  +2/1 -> r/1
  x6/1 -> r2/1, Mux/2
  s/1 -> +2/2
  r2/1 -> +2/1
  Mux/1 -> s/1

== system test_TFOIDFF/TFOIDFFID/ITAE/Subsystem/TRAS 2_dof model 3/DCP-azimuth ==
  CTR_A : Inport
  1/Ja : Gain  Gain=37000  SaturateOnIntegerOverflow=on  OutDataTypeStr=Inherit: Same as input  ParamDataTypeStr=Inherit: Same as input
  CtrlA(rpma) : Lookup  InputValues=rpm_a  Table=control_a
  Integrator1 : Integrator
  Sum1 : Sum  Inputs=|+-  InputSameDT=on  SaturateOnIntegerOverflow=on  OutDataTypeStr=Inherit: Same as first input
  forceA(rpma) : Lookup  InputValues=rpm_a  Table=force_a
  RPM_A : Outport
  FORCE_A : Outport  Port=2
  wires:
  Sum1/1 -> Integrator1/1
  CtrlA(rpma)/1 -> Sum1/2
  Integrator1/1 -> 1/Ja/1
  1/Ja/1 -> CtrlA(rpma)/1, forceA(rpma)/1, RPM_A/1
  CTR_A/1 -> Sum1/1
  forceA(rpma)/1 -> FORCE_A/1

== system test_TFOIDFF/TFOIDFFID/ITAE/Subsystem/TRAS 2_dof model 3/DCP_pith ==
  CTR_P : Inport
  1/Jp1 : Gain  Gain=6100  OutDataTypeStr=Inherit: Same as input  ParamDataTypeStr=Inherit: Same as input
  CtrlP(rpmp) : Lookup  InputValues=rpm_p  Table=control_p
  Integrator : Integrator
  Sum : Sum  Inputs=|+-  InputSameDT=on  SaturateOnIntegerOverflow=on  OutDataTypeStr=Inherit: Same as first input
  force(rpmp) : Lookup  InputValues=rpm_p  Table=force_p
  RPM_P : Outport
  FORCE_P : Outport  Port=2
  wires:
  Sum/1 -> Integrator/1
  Integrator/1 -> 1/Jp1/1
  CtrlP(rpmp)/1 -> Sum/2
  1/Jp1/1 -> RPM_P/1, CtrlP(rpmp)/1, force(rpmp)/1
  CTR_P/1 -> Sum/1
  force(rpmp)/1 -> FORCE_P/1

== system test_TFOIDFF/TFOIDFFID/ITAE/Subsystem/TRAS 2_dof model 3/q (x2,x6) ==
  x2 : Inport
  x6 : Inport  Port=2
  " q(x6)" : Fcn  Expr=( (0.0268-0.00300962066650)*cos(u)^2) +0.00300962066650
  *1 : Product  Inputs=*/  InputSameDT=on  SaturateOnIntegerOverflow=on  OutDataTypeStr=Inherit: Same as first input
  q : Outport
  wires:
  *1/1 -> q/1
  x2/1 -> *1/1
  x6/1 -> " q(x6)"/1
  " q(x6)"/1 -> *1/2

== system test_TFOIDFF/TFOIDFFID/ITAE/Subsystem/TRAS 2_dof model 3/r(x2,x6) ==
  y2 : Inport
  x6 : Inport  Port=2
  +2 : Sum  InputSameDT=on  SaturateOnIntegerOverflow=on  OutDataTypeStr=Inherit: Same as first input
  Mux : Mux  Inputs=2
  r2 : Fcn  Expr=- ( 0.0292*cos(u)+ 0.0546*sin(u))*1.7143
  s : Fcn  Expr="(u(1)^2)*(     -0.07389953104162*  0.28753198180218*sin(u(2))*cos(u(2)))"
  r : Outport
  wires:
  Mux/1 -> s/1
  r2/1 -> +2/1
  s/1 -> +2/2
  x6/1 -> Mux/2, r2/1
  +2/1 -> r/1
  y2/1 -> Mux/1

== system test_TFOIDFF/TFOIDFFID/ITSE/Subsystem/TRAS 2_dof model 3/DCP-azimuth ==
  CTR_A : Inport
  1/Ja : Gain  Gain=37000  SaturateOnIntegerOverflow=on  OutDataTypeStr=Inherit: Same as input  ParamDataTypeStr=Inherit: Same as input
  CtrlA(rpma) : Lookup  InputValues=rpm_a  Table=control_a
  Integrator1 : Integrator
  Sum1 : Sum  Inputs=|+-  InputSameDT=on  SaturateOnIntegerOverflow=on  OutDataTypeStr=Inherit: Same as first input
  forceA(rpma) : Lookup  InputValues=rpm_a  Table=force_a
  RPM_A : Outport
  FORCE_A : Outport  Port=2
  wires:
  Sum1/1 -> Integrator1/1
  CtrlA(rpma)/1 -> Sum1/2
  Integrator1/1 -> 1/Ja/1
  1/Ja/1 -> CtrlA(rpma)/1, forceA(rpma)/1, RPM_A/1
  CTR_A/1 -> Sum1/1
  forceA(rpma)/1 -> FORCE_A/1

== system test_TFOIDFF/TFOIDFFID/ITSE/Subsystem/TRAS 2_dof model 3/DCP_pith ==
  CTR_P : Inport
  1/Jp1 : Gain  Gain=6100  OutDataTypeStr=Inherit: Same as input  ParamDataTypeStr=Inherit: Same as input
  CtrlP(rpmp) : Lookup  InputValues=rpm_p  Table=control_p
  Integrator : Integrator
  Sum : Sum  Inputs=|+-  InputSameDT=on  SaturateOnIntegerOverflow=on  OutDataTypeStr=Inherit: Same as first input
  force(rpmp) : Lookup  InputValues=rpm_p  Table=force_p
  RPM_P : Outport
  FORCE_P : Outport  Port=2
  wires:
  Sum/1 -> Integrator/1
  Integrator/1 -> 1/Jp1/1
  CtrlP(rpmp)/1 -> Sum/2
  1/Jp1/1 -> RPM_P/1, CtrlP(rpmp)/1, force(rpmp)/1
  CTR_P/1 -> Sum/1
  force(rpmp)/1 -> FORCE_P/1

== system test_TFOIDFF/TFOIDFFID/ITSE/Subsystem/TRAS 2_dof model 3/q (x2,x6) ==
  x2 : Inport
  x6 : Inport  Port=2
  " q(x6)" : Fcn  Expr=( (0.0268-0.00300962066650)*cos(u)^2) +0.00300962066650
  *1 : Product  Inputs=*/  InputSameDT=on  SaturateOnIntegerOverflow=on  OutDataTypeStr=Inherit: Same as first input
  q : Outport
  wires:
  *1/1 -> q/1
  x2/1 -> *1/1
  x6/1 -> " q(x6)"/1
  " q(x6)"/1 -> *1/2

== system test_TFOIDFF/TFOIDFFID/ITSE/Subsystem/TRAS 2_dof model 3/r(x2,x6) ==
  y2 : Inport
  x6 : Inport  Port=2
  +2 : Sum  InputSameDT=on  SaturateOnIntegerOverflow=on  OutDataTypeStr=Inherit: Same as first input
  Mux : Mux  Inputs=2
  r2 : Fcn  Expr=- ( 0.0292*cos(u)+ 0.0546*sin(u))*1.7143
  s : Fcn  Expr="(u(1)^2)*(     -0.07389953104162*  0.28753198180218*sin(u(2))*cos(u(2)))"
  r : Outport
  wires:
  Mux/1 -> s/1
  r2/1 -> +2/1
  s/1 -> +2/2
  x6/1 -> Mux/2, r2/1
  +2/1 -> r/1
  y2/1 -> Mux/1

== system test_TFOIDFF/TFOIDFFID/sensibility/Subsystem/TRAS 2_dof model 3/DCP-azimuth ==
  CTR_A : Inport
  1/Ja : Gain  Gain=37000  SaturateOnIntegerOverflow=on  OutDataTypeStr=Inherit: Same as input  ParamDataTypeStr=Inherit: Same as input
  CtrlA(rpma) : Lookup  InputValues=rpm_a  Table=control_a
  Integrator1 : Integrator
  Sum1 : Sum  Inputs=|+-  InputSameDT=on  SaturateOnIntegerOverflow=on  OutDataTypeStr=Inherit: Same as first input
  forceA(rpma) : Lookup  InputValues=rpm_a  Table=force_a
  RPM_A : Outport
  FORCE_A : Outport  Port=2
  wires:
  forceA(rpma)/1 -> FORCE_A/1
  CTR_A/1 -> Sum1/1
  1/Ja/1 -> RPM_A/1, forceA(rpma)/1, CtrlA(rpma)/1
  Integrator1/1 -> 1/Ja/1
  CtrlA(rpma)/1 -> Sum1/2
  Sum1/1 -> Integrator1/1

== system test_TFOIDFF/TFOIDFFID/sensibility/Subsystem/TRAS 2_dof model 3/DCP_pith ==
  CTR_P : Inport
  1/Jp1 : Gain  Gain=6100  OutDataTypeStr=Inherit: Same as input  ParamDataTypeStr=Inherit: Same as input
  CtrlP(rpmp) : Lookup  InputValues=rpm_p  Table=control_p
  Integrator : Integrator
  Sum : Sum  Inputs=|+-  InputSameDT=on  SaturateOnIntegerOverflow=on  OutDataTypeStr=Inherit: Same as first input
  force(rpmp) : Lookup  InputValues=rpm_p  Table=force_p
  RPM_P : Outport
  FORCE_P : Outport  Port=2
  wires:
  force(rpmp)/1 -> FORCE_P/1
  CTR_P/1 -> Sum/1
  1/Jp1/1 -> force(rpmp)/1, CtrlP(rpmp)/1, RPM_P/1
  CtrlP(rpmp)/1 -> Sum/2
  Integrator/1 -> 1/Jp1/1
  Sum/1 -> Integrator/1

== system test_TFOIDFF/TFOIDFFID/sensibility/Subsystem/TRAS 2_dof model 3/q (x2,x6) ==
  x2 : Inport
  x6 : Inport  Port=2
  " q(x6)" : Fcn  Expr=( (0.0268-0.00300962066650)*cos(u)^2) +0.00300962066650
  *1 : Product  Inputs=*/  InputSameDT=on  SaturateOnIntegerOverflow=on  OutDataTypeStr=Inherit: Same as first input
  q : Outport
  wires:
  " q(x6)"/1 -> *1/2
  x6/1 -> " q(x6)"/1
  x2/1 -> *1/1
  *1/1 -> q/1

== system test_TFOIDFF/TFOIDFFID/sensibility/Subsystem/TRAS 2_dof model 3/r(x2,x6) ==
  y2 : Inport
  x6 : Inport  Port=2
  +2 : Sum  InputSameDT=on  SaturateOnIntegerOverflow=on  OutDataTypeStr=Inherit: Same as first input
  Mux : Mux  Inputs=2
  r2 : Fcn  Expr=- ( 0.0292*cos(u)+ 0.0546*sin(u))*1.7143
  s : Fcn  Expr="(u(1)^2)*(     -0.07389953104162*  0.28753198180218*sin(u(2))*cos(u(2)))"
  r : Outport
  wires:
  y2/1 -> Mux/1
  +2/1 -> r/1
  x6/1 -> r2/1, Mux/2
  s/1 -> +2/2
  r2/1 -> +2/1
  Mux/1 -> s/1
